simulink subsystem "sensor_imu"  (R2026a)
settings: Solver=VariableStepAuto
model mask{samplingrate=500, noise_accel=[1,1,1]*1e-3, bias_accel=[0 0 0], scale_accel=[1 0 0; 0 1 0; 0 0 1], lim_accel=inf, noise_gyro=[1,1,1]*1e-9, bias_gyro=[0 0 0], scale_gyro=[1 0 0; 0 1 0; 0 0 1], lim_gyro=inf, S=[1 0 0; 0 1 0; 0 0 1], d=[0 0 0]}
  mask prompts: samplingrate "Sampling Time (s)"; noise_accel "Accelerometer Noise Power"; bias_accel "Accelerometer Bias"; scale_accel "Accelerometer Scaling"; lim_accel "Accelerometer Limit"; noise_gyro "Gyro Noise Power"; bias_gyro "Gyro Bias"; scale_gyro "Gyro Scaling"; lim_gyro "Gyro Limit"; S "Body to Sensor rotation"; d "Sensor Location in Body frame"
libraries: aerolibnav x1
settings Model: Creator=finnb  LastModifiedBy=trist

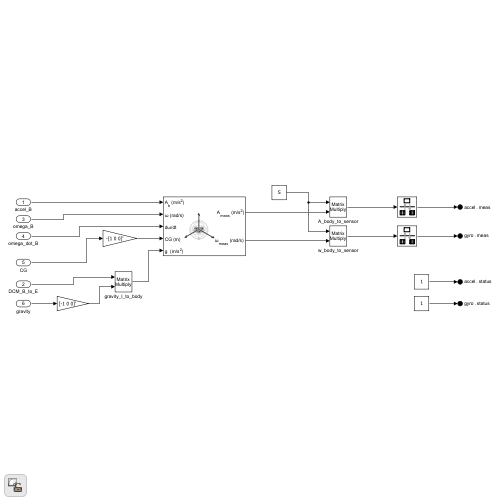
[thumbnail: Simulink's stored preview of the top-level diagram]
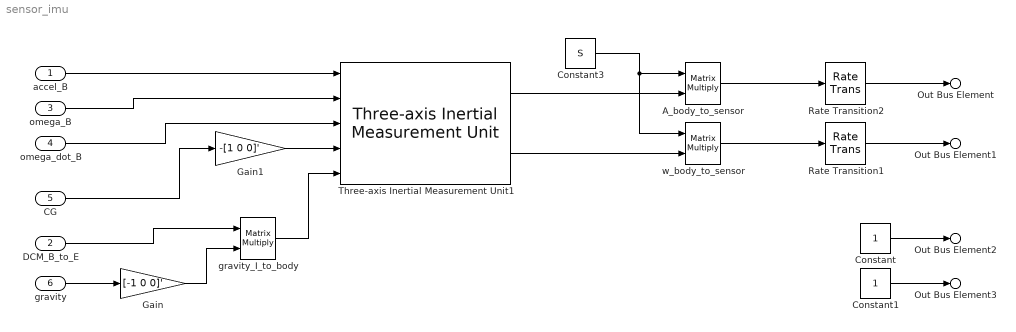
== system sensor_imu ==
  accel_B : Inport
  DCM_B_to_E : Inport  Port=2
  omega_B : Inport  Port=3
  omega_dot_B : Inport  Port=4
  CG : Inport  Port=5
  gravity : Inport  Port=6
  A_body_to_sensor : Product  Multiplication=Matrix(*)
  Constant : Constant  OutDataTypeStr=boolean
  Constant1 : Constant  OutDataTypeStr=boolean
  Constant3 : Constant  Value=S
  Gain : Gain  Gain=[-1 0 0]'
  Gain1 : Gain  Gain=-[1 0 0]'
  Rate Transition1 : RateTransition  OutPortSampleTime=samplingrate
  Rate Transition2 : RateTransition  OutPortSampleTime=samplingrate
  Three-axis Inertial Measurement Unit1 : aerolibnav/Three-axis Inertial Measurement Unit  units=Metric (MKS)  imu=-d  i_Ts=samplingrate  dtype_a=off  w_a=190  z_a=0.707  a_sf_cc=scale_accel  a_bias="bias_accel  .* (2*rand(1,3)-1)"  a_sat="[-lim_accel  -lim_accel  -lim_accel  lim_accel lim_accel lim_accel]"  dtype_g=off  w_g=190  z_g=0.707  g_sf_cc=scale_gyro  g_bias="bias_gyro  .* (2*rand(1,3)-1)"  g_sens=[0 0 0]  g_sat="[-lim_gyro  -lim_gyro  -lim_gyro lim_gyro lim_gyro lim_gyro]"  i_rand=on  i_seeds=[23093 23094 23095 23096 23097 23098]  i_pow="[noise_accel,  noise_gyro]"
  gravity_I_to_body : Product  Multiplication=Matrix(*)
  w_body_to_sensor : Product  Multiplication=Matrix(*)
  Out Bus Element : Outport  PortName=accel  Element=meas
  Out Bus Element2 : Outport  PortName=accel  Element=status
  Out Bus Element1 : Outport  Port=2  PortName=gyro  Element=meas
  Out Bus Element3 : Outport  Port=2  PortName=gyro  Element=status
  wires:
  accel_B/1 -> Three-axis Inertial Measurement Unit1/1
  omega_B/1 -> Three-axis Inertial Measurement Unit1/2
  omega_dot_B/1 -> Three-axis Inertial Measurement Unit1/3
  gravity_I_to_body/1 -> Three-axis Inertial Measurement Unit1/5
  Constant3/1 -> w_body_to_sensor/1, A_body_to_sensor/1
  w_body_to_sensor/1 -> Rate Transition1/1
  Gain/1 -> gravity_I_to_body/2
  gravity/1 -> Gain/1
  DCM_B_to_E/1 -> gravity_I_to_body/1
  Three-axis Inertial Measurement Unit1/1 -> A_body_to_sensor/2
  Three-axis Inertial Measurement Unit1/2 -> w_body_to_sensor/2
  Rate Transition1/1 -> Out Bus Element1/1
  A_body_to_sensor/1 -> Rate Transition2/1
  Rate Transition2/1 -> Out Bus Element/1
  Constant/1 -> Out Bus Element2/1
  Constant1/1 -> Out Bus Element3/1
  CG/1 -> Gain1/1
  Gain1/1 -> Three-axis Inertial Measurement Unit1/4
